simulink library "Gravity_Lib"  (R2016b)
settings: Solver=ode45  StartTime=0.0  StopTime=10.0  RelTol=1e-3
values from neighbouring files (symbols this model uses):
  AC = miniMUTT_config    [UAV_config.m]
libraries: simulink x1
settings Model: Creator=Paul Freeman  LastModifiedBy=UAVLAB
settings DataIOCC: LimitDataPoints=on  SaveFormat=Array  SignalLoggingSaveFormat=ModelDataLogs
settings OptimizationCC: BlockReduction=off  BooleanDataType=off  ExpressionDepthLimit=2147483647  LifeSpan=inf
settings DebuggingCC: SaveWithParameterizedLinksMsg=none  UnderspecifiedInitializationDetection=Classic  MergeDetectMultiDrivingBlocksExec=none  SignalResolutionControl=TryResolveAllWithWarning  FcnCallInpInsideContextMsg=warning  StateNameClashWarn=warning  StrictBusMsg=Warning  SFUnexpectedBacktrackingDiag=warning  SFNoUnconditionalDefaultTransitionDiag=warning  SFExecutionAtInitializationDiag=none
settings HardwareCC: ProdBitPerPointer=32  ProdBitPerSizeT=32  ProdBitPerPtrDiffT=32  ProdLargestAtomicFloat=None  ProdIntDivRoundTo=Undefined  ProdEndianess=Unspecified  ProdWordSize=32  ProdHWDeviceType=32-bit Generic  TargetUnknown=on
settings ModelReferenceCC: PropagateSignalLabelsOutOfModel=off
settings GRTTargetCC: TargetLangStandard=C89/C90 (ANSI)  GeneratePreprocessorConditionals=Disable all  CombineOutputUpdateFcns=off  GRTInterface=on
settings ConfigComp: CovMetricSettings=dw  CovHtmlReporting=on  CovSaveCumulativeToWorkspaceVar=on  CovSaveSingleToWorkspaceVar=on  CovExternalEMLEnable=off

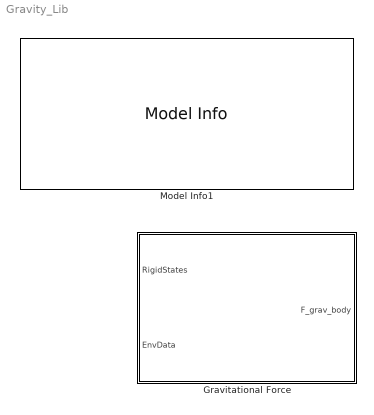
== system Gravity_Lib ==
  "Gravitational Force " : Subsystem
  Model Info1 : simulink/Model-Wide Utilities/Model Info  BlockCM=None  Frame=on  DisplayStringWithTags=|  HorizontalTextAlignment=Left  LeftAlignmentValue=0.02  SourceBlockDiagram=Gravity_Lib  TagMaxNumber=20
      | MODEL INFORMATION
      | Gravitational Force Library
      | 
      | University of Minnesota
      | Aerospace Engineering and Mechanics
      | Copyright 2011 Regents of the University of Minnesota. All rights reserved.
      | 
      | == SVN Info ==
      | %<ModelVersion>
      | Last modified by %<LastModifiedBy> on %<LastModificationDate>

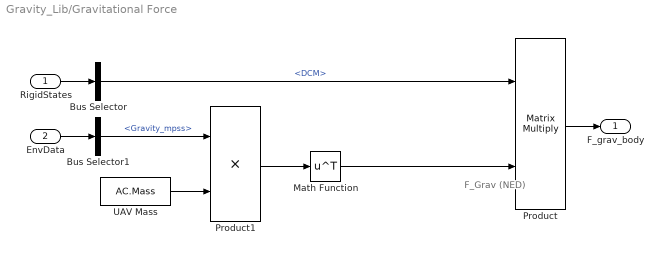
== system Gravity_Lib/Gravitational Force  ==
  note: F_Grav (NED)
  RigidStates : Inport  OutDataTypeStr=Bus: RigidStates
  EnvData : Inport  Port=2  OutDataTypeStr=Bus: EnvData
  Bus Selector : BusSelector  OutputSignals=DCM
  Bus Selector1 : BusSelector  OutputSignals=Gravity_mpss
  Math Function : Math  Operator=transpose  SaturateOnIntegerOverflow=on
  Product : Product  Multiplication=Matrix(*)  SaturateOnIntegerOverflow=on  RndMeth=Zero  InputSameDT=on  OutDataTypeStr=Inherit: Same as first input
  Product1 : Product  SaturateOnIntegerOverflow=on  RndMeth=Zero  InputSameDT=on  OutDataTypeStr=Inherit: Same as first input
  UAV Mass : Constant  Value=AC.Mass
  F_grav_body : Outport
  wires:
  Product/1 -> F_grav_body/1
  Bus Selector/1 -> Product/1  "<DCM>"
  RigidStates/1 -> Bus Selector/1
  EnvData/1 -> Bus Selector1/1
  Bus Selector1/1 -> Product1/1  "<Gravity_mpss>"
  UAV Mass/1 -> Product1/2
  Product1/1 -> Math Function/1
  Math Function/1 -> Product/2
